simulink model "MI_T1_REF"  (R2023b)
settings: Solver=FixedStepDiscrete  StartTime=0.0  StopTime=10.0  FixedStep=0.01  RelTol=1e-3
settings Model: DataDictionary=BMS_MAIN.sldd  Creator=Somashekar M  LastModifiedBy=Somashekar M

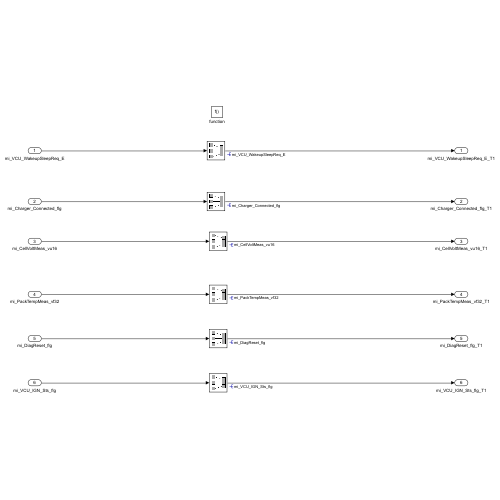
[thumbnail: Simulink's stored preview of the top-level diagram]
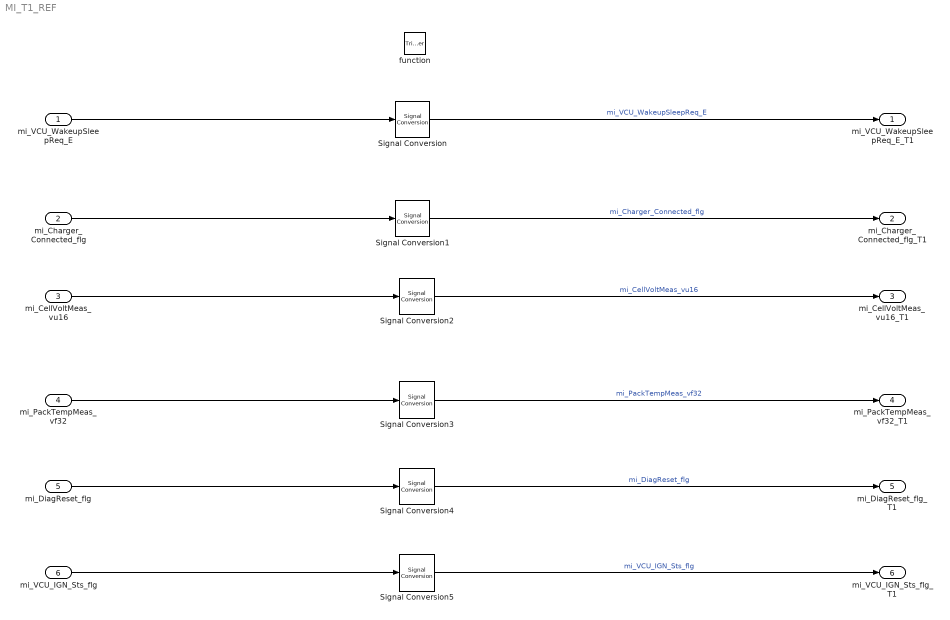
== system MI_T1_REF ==
  mi_VCU_WakeupSleepReq_E : Inport
  mi_Charger_Connected_flg : Inport  Port=2
  mi_CellVoltMeas_vu16 : Inport  Port=3
  mi_PackTempMeas_vf32 : Inport  Port=4
  mi_DiagReset_flg : Inport  Port=5
  mi_VCU_IGN_Sts_flg : Inport  Port=6
  function : TriggerPort  TriggerType=function-call  VariantControl=(inherit)
  Signal Conversion{,1..5} (6 alike) : SignalConversion  OverrideOpt=off
  mi_VCU_WakeupSleepReq_E_T1 : Outport
  mi_Charger_Connected_flg_T1 : Outport  Port=2
  mi_CellVoltMeas_vu16_T1 : Outport  Port=3
  mi_PackTempMeas_vf32_T1 : Outport  Port=4
  mi_DiagReset_flg_T1 : Outport  Port=5
  mi_VCU_IGN_Sts_flg_T1 : Outport  Port=6
  wires:
  Signal Conversion/1 -> mi_VCU_WakeupSleepReq_E_T1/1  "mi_VCU_WakeupSleepReq_E"
  mi_Charger_Connected_flg/1 -> Signal Conversion1/1
  mi_CellVoltMeas_vu16/1 -> Signal Conversion2/1
  mi_PackTempMeas_vf32/1 -> Signal Conversion3/1
  mi_DiagReset_flg/1 -> Signal Conversion4/1
  mi_VCU_IGN_Sts_flg/1 -> Signal Conversion5/1
  mi_VCU_WakeupSleepReq_E/1 -> Signal Conversion/1
  Signal Conversion1/1 -> mi_Charger_Connected_flg_T1/1  "mi_Charger_Connected_flg"
  Signal Conversion3/1 -> mi_PackTempMeas_vf32_T1/1  "mi_PackTempMeas_vf32"
  Signal Conversion4/1 -> mi_DiagReset_flg_T1/1  "mi_DiagReset_flg"
  Signal Conversion5/1 -> mi_VCU_IGN_Sts_flg_T1/1  "mi_VCU_IGN_Sts_flg"
  Signal Conversion2/1 -> mi_CellVoltMeas_vu16_T1/1  "mi_CellVoltMeas_vu16"
